simulink model "Australian14gen_forming_inertia"  (R2017b)
(part 2 of 4)

  T8/LConn2 -- B301/RConn2
  T8/RConn1 -- B303/LConn1
  T8/RConn2 -- B303/LConn2
  T8/RConn3 -- B303/LConn3
  B304/RConn1 -- L-23/LConn1 -- T10/LConn1
  B304/RConn2 -- L-23/LConn2 -- T10/LConn2
  T10/LConn3 -- L-23/LConn3 -- B304/RConn3
  L-33/LConn1 -- B314/RConn1
  L-33/LConn2 -- B314/RConn2
  L-33/LConn3 -- B314/RConn3
  L-33/RConn1 -- B313/LConn1
  L-33/RConn2 -- B313/LConn2
  L-33/RConn3 -- B313/LConn3
  T12/RConn3 -- Load17/LConn3 -- T22/RConn3 -- B314/LConn3
  T12/RConn2 -- T22/RConn2 -- Load17/LConn2 -- B314/LConn2
  T12/RConn1 -- T22/RConn1 -- Load17/LConn1 -- B314/LConn1
  T10/RConn1 -- B313/RConn1 -- Load16/LConn1 -- L-32/LConn1
  B313/RConn2 -- Load16/LConn2 -- L-32/LConn2 -- T10/RConn2
  T10/RConn3 -- B313/RConn3 -- Load16/LConn3 -- L-32/LConn3
  B312/LConn2 -- Load15/LConn2 -- L-32/RConn2
  L-32/RConn1 -- Load15/LConn1 -- B312/LConn1
  L-32/RConn3 -- Load15/LConn3 -- B312/LConn3
  G302_YPS/LConn3 -- B302/LConn3 -- Load Flow Bus11/LConn1
  T9/LConn3 -- B302/RConn3
  B312/RConn3 -- T18/RConn3 -- T9/RConn3
  T9/LConn2 -- B302/RConn2
  T9/LConn1 -- B302/RConn1
  B312/RConn2 -- T18/RConn2 -- T9/RConn2
  G302_YPS/LConn1 -- B302/LConn1
  G302_YPS/LConn2 -- B302/LConn2
  B312/RConn1 -- T18/RConn1 -- T9/RConn1
  B306/RConn1 -- L-26/LConn1 -- Load11/LConn1
  L-26/LConn2 -- Load11/LConn2 -- B306/RConn2
  B306/RConn3 -- L-26/LConn3 -- Load11/LConn3
  L-28/RConn1 -- B306/LConn1
  L-28/RConn2 -- B306/LConn2
  L-28/RConn3 -- B306/LConn3
  T11/RConn1 -- B311/LConn1
  T11/RConn2 -- B311/LConn2
  T11/RConn3 -- B311/LConn3
  B308/LConn1 -- Load13/LConn1 -- T13/LConn1
  B308/LConn2 -- Load13/LConn2 -- T13/LConn2
  B308/LConn3 -- Load13/LConn3 -- T13/LConn3
  T13/RConn1 -- B315/LConn1
  T13/RConn2 -- B315/LConn2
  T13/RConn3 -- B315/LConn3
  L-49-2/LConn1 -- B504/LConn1 -- L-48-1/LConn1 -- L-48-2/LConn1 -- L-49-1/LConn1
  L-49-2/LConn2 -- L-49-1/LConn2 -- L-48-1/LConn2 -- B504/LConn2 -- L-48-2/LConn2
  L-49-2/LConn3 -- L-49-1/LConn3 -- B504/LConn3 -- L-48-1/LConn3 -- L-48-2/LConn3
  B507/RConn2 -- Load27/LConn2 -- L-50-1/LConn2 -- L-48-2/RConn2 -- L-48-1/RConn2
  B507/RConn1 -- Load27/LConn1 -- L-48-2/RConn1 -- L-48-1/RConn1 -- L-50-1/LConn1
  B507/RConn3 -- Load27/LConn3 -- L-48-2/RConn3 -- L-48-1/RConn3 -- L-50-1/LConn3
  B509/RConn1 -- L-55-2/RConn1 -- L-55-1/RConn1
  B509/RConn2 -- L-55-2/RConn2 -- L-55-1/RConn2
  B509/RConn3 -- L-55-2/RConn3 -- L-55-1/RConn3
  L-55-2/LConn1 -- L-54/LConn1 -- L-55-1/LConn1 -- L-52/LConn1 -- B507/LConn1
  B507/LConn2 -- L-55-1/LConn2 -- L-52/LConn2 -- L-54/LConn2 -- L-55-2/LConn2
  L-54/LConn3 -- L-55-2/LConn3 -- B507/LConn3 -- L-55-1/LConn3 -- L-52/LConn3
  L-34-1/RConn1 -- L-34-2/RConn1 -- Three-Phase V-I Measurement4/RConn1
  L-34-1/RConn2 -- L-34-2/RConn2 -- Three-Phase V-I Measurement4/RConn2
  L-34-1/RConn3 -- L-34-2/RConn3 -- Three-Phase V-I Measurement4/RConn3
  B509/LConn1 -- Load29/LConn1 -- L-34-1/LConn1 -- L-34-2/LConn1
  Load29/LConn2 -- L-34-2/LConn2 -- L-34-1/LConn2 -- B509/LConn2
  B509/LConn3 -- L-34-1/LConn3 -- Load29/LConn3 -- L-34-2/LConn3
  G503_PPS/LConn3 -- Load Flow Bus12/LConn1 -- B503/LConn3
  G503_PPS/LConn1 -- B503/LConn1
  B503/RConn2 -- T21/LConn2
  B503/RConn3 -- T21/LConn3
  B503/RConn1 -- T21/LConn1
  G503_PPS/LConn2 -- B503/LConn2
  B506/RConn1 -- L-53/RConn1 -- L-52/RConn1
  B506/RConn2 -- L-53/RConn2 -- L-52/RConn2
  B506/RConn3 -- L-53/RConn3 -- L-52/RConn3
  B506/LConn2 -- T21/RConn2
  B506/LConn3 -- T21/RConn3
  B506/LConn1 -- T21/RConn1
  L-49-2/RConn1 -- L-49-1/RConn1 -- L-51/RConn1 -- L-54/RConn1 -- L-53/LConn1 -- B508/RConn1
  L-49-2/RConn2 -- L-49-1/RConn2 -- L-51/RConn2 -- L-54/RConn2 -- L-53/LConn2 -- B508/RConn2
  L-49-2/RConn3 -- L-49-1/RConn3 -- L-51/RConn3 -- L-54/RConn3 -- L-53/LConn3 -- B508/RConn3
  Load28/LConn1 -- T40/RConn1 -- T24/RConn1 -- B508/LConn1
  Load28/LConn2 -- T24/RConn2 -- T40/RConn2 -- B508/LConn2
  Load28/LConn3 -- T40/RConn3 -- T24/RConn3 -- B508/LConn3
  B505/RConn1 -- L-51/LConn1 -- L-50-1/RConn1
  B505/RConn2 -- L-51/LConn2 -- L-50-1/RConn2
  B505/RConn3 -- L-51/LConn3 -- L-50-1/RConn3
  B505/LConn3 -- T34/RConn3 -- T20/RConn3
  B502/RConn2 -- T20/LConn2
  B502/RConn1 -- T20/LConn1
  B505/LConn2 -- T34/RConn2 -- T20/RConn2
  B502/RConn3 -- T20/LConn3
  B505/LConn1 -- T34/RConn1 -- T20/RConn1
  B501/LConn2 -- T19/LConn2
  B501/LConn3 -- T19/LConn3
  B501/LConn1 -- T19/LConn1
  B504/RConn2 -- Load26/LConn2 -- T25/RConn2 -- T19/RConn2
  B504/RConn1 -- Load26/LConn1 -- T25/RConn1 -- T19/RConn1
  B504/RConn3 -- Load26/LConn3 -- T19/RConn3 -- T25/RConn3
  Load19/LConn1 -- B406/LConn1
  Load19/LConn2 -- B406/LConn2
  Load19/LConn3 -- B406/LConn3
  B204/LConn3 -- T5/LConn3
  G204_MPS/LConn1 -- Load Flow Bus8/LConn1 -- B204/RConn1
  G204_MPS/LConn3 -- B204/RConn3
  G204_MPS/LConn2 -- B204/RConn2
  B204/LConn1 -- T5/LConn1
  B204/LConn2 -- T5/LConn2
  B415/LConn1 -- Comp7-415/LConn1 -- L-47-2/LConn1 -- L-47-1/LConn1
  B415/LConn2 -- Comp7-415/LConn2 -- L-47-2/LConn2 -- L-47-1/LConn2
  B415/LConn3 -- Comp7-415/LConn3 -- L-47-2/LConn3 -- L-47-1/LConn3
  B416/RConn2 -- L-47-1/RConn2 -- L-47-2/RConn2
  B416/RConn3 -- L-47-1/RConn3 -- L-47-2/RConn3
  B416/RConn1 -- L-47-1/RConn1 -- L-47-2/RConn1
  B308/RConn1 -- T23/RConn1 -- L-29-1/LConn1 -- L-29-2/LConn1
  B308/RConn2 -- T23/RConn2 -- L-29-1/LConn2 -- L-29-2/LConn2
  B308/RConn3 -- T23/RConn3 -- L-29-1/LConn3 -- L-29-2/LConn3
  B307/LConn1 -- Load12/LConn1 -- L-29-1/RConn1 -- L-29-2/RConn1
  B307/LConn2 -- Load12/LConn2 -- L-29-1/RConn2 -- L-29-2/RConn2
  B307/LConn3 -- Load12/LConn3 -- L-29-1/RConn3 -- L-29-2/RConn3
  B205/RConn3 -- Three-Phase V-I Measurement1/RConn3
  B205/RConn2 -- Three-Phase V-I Measurement1/RConn2
  B205/RConn1 -- Three-Phase V-I Measurement1/RConn1
  L-30-2/LConn1 -- L-30-1/LConn1 -- B309/LConn1 -- Load14/LConn1
  2/RConn1 -- B310/LConn1 -- 1/RConn1
  1/RConn2 -- 2/RConn2 -- B310/LConn2
  2/RConn3 -- B310/LConn3 -- 1/RConn3
  2/LConn1 -- B311/RConn1 -- 1/LConn1
  2/LConn2 -- B311/RConn2 -- 1/LConn2
  1/LConn3 -- 2/LConn3 -- B311/RConn3
  L-2-1/RConn2 -- L-1-1/RConn2 -- L-1-2/RConn2 -- Three-Phase V-I Measurement2/LConn2 -- L-2-2/RConn2
  B102/RConn1 -- T27/RConn1 -- Three-Phase V-I Measurement2/RConn1
  B102/RConn2 -- T27/RConn2 -- Three-Phase V-I Measurement2/RConn2
  B102/RConn3 -- T27/RConn3 -- Three-Phase V-I Measurement2/RConn3
  L-30-1/RConn1 -- L-30-2/RConn1 -- B310/RConn1
  L-30-1/RConn2 -- L-30-2/RConn2 -- B310/RConn2
  L-30-1/RConn3 -- L-30-2/RConn3 -- B310/RConn3
  Three-Phase V-I Measurement3/RConn1 -- T26/RConn1 -- B309/RConn1
  Three-Phase V-I Measurement3/RConn2 -- T26/RConn2 -- B309/RConn2
  Three-Phase V-I Measurement3/RConn3 -- T26/RConn3 -- B309/RConn3
  B315/RConn3 -- Three-Phase V-I Measurement4/LConn3
  B315/RConn2 -- Three-Phase V-I Measurement4/LConn2
  B315/RConn1 -- Three-Phase V-I Measurement4/LConn1
  G404_GPS/LConn2 -- B404/RConn2
  G404_GPS/LConn1 -- B404/RConn1
  CPS403/LConn2 -- 20kV 2000MVA14/RConn2 -- 20kV 2000MVA1/RConn2 -- B403_vi/LConn2
  CPS403/LConn1 -- 20kV 2000MVA14/RConn1 -- 20kV 2000MVA1/RConn1 -- B403_vi/LConn1
  B402/LConn2 -- CPS402/LConn2
  CPS402/LConn3 -- B402/LConn3
  Load Flow Bus13/LConn1 -- 3-Phase Dynamic Load3/LConn3 -- B502/LConn3
  G501_NPS/LConn1 -- B501/RConn1
  B501/RConn2 -- G501_NPS/LConn2
  G501_NPS/LConn3 -- Load Flow Bus14/LConn1 -- B501/RConn3
  20kV 2000MVA8/RConn1 -- B312_vi/RConn1 -- 20kV 2000MVA19/RConn1
  20kV 2000MVA8/RConn2 -- B312_vi/RConn2 -- 20kV 2000MVA19/RConn2
  20kV 2000MVA8/RConn3 -- 20kV 2000MVA19/RConn3 -- B312_vi/RConn3
  B312_vi/LConn3 -- T18/LConn3
  T18/LConn2 -- B312_vi/LConn2
  T18/LConn1 -- B312_vi/LConn1
  B314_vi/LConn3 -- T22/LConn3
  20kV 2000MVA7/RConn2 -- 20kV 2000MVA20/RConn2 -- B314_vi/RConn2
  T22/LConn1 -- B314_vi/LConn1
  T22/LConn2 -- B314_vi/LConn2
  20kV 2000MVA7/RConn1 -- 20kV 2000MVA20/RConn1 -- B314_vi/RConn1
  20kV 2000MVA7/RConn3 -- 20kV 2000MVA20/RConn3 -- B314_vi/RConn3
  20kV 2000MVA10/RConn2 -- 20kV 2000MVA24/RConn2 -- B308_vi/LConn2
  T23/LConn2 -- B308_vi/RConn2
  T23/LConn3 -- B308_vi/RConn3
  20kV 2000MVA10/RConn1 -- 20kV 2000MVA24/RConn1 -- B308_vi/LConn1
  T23/LConn1 -- B308_vi/RConn1
  20kV 2000MVA10/RConn3 -- 20kV 2000MVA24/RConn3 -- B308_vi/LConn3
  B508_vi/LConn3 -- 20kV 2000MVA26/RConn1 -- 20kV 2000MVA13/RConn1
  B508_vi/LConn2 -- 20kV 2000MVA26/RConn2 -- 20kV 2000MVA13/RConn2
  B508_vi/LConn1 -- 20kV 2000MVA26/RConn3 -- 20kV 2000MVA13/RConn3
  T25/LConn3 -- B504_vi/RConn3
  T25/LConn1 -- B504_vi/RConn1
  T25/LConn2 -- B504_vi/RConn2
  20kV 2000MVA11/RConn1 -- 20kV 2000MVA27/RConn1 -- B504_vi/LConn1
  20kV 2000MVA11/RConn2 -- 20kV 2000MVA27/RConn2 -- B504_vi/LConn2
  20kV 2000MVA11/RConn3 -- 20kV 2000MVA27/RConn3 -- B504_vi/LConn3
  B508_vi/RConn3 -- T24/LConn1
  T24/LConn2 -- B508_vi/RConn2
  B508_vi/RConn1 -- T24/LConn3
  20kV 2000MVA9/RConn1 -- 20kV 2000MVA25/RConn1 -- B309_vi/RConn3
  20kV 2000MVA9/RConn2 -- 20kV 2000MVA25/RConn2 -- B309_vi/RConn2
  20kV 2000MVA9/RConn3 -- 20kV 2000MVA25/RConn3 -- B309_vi/RConn1
  T26/LConn1 -- B309_vi/LConn3
  T26/LConn2 -- B309_vi/LConn2
  T26/LConn3 -- B309_vi/LConn1
  B102_vi/LConn1 -- T27/LConn1
  B102_vi/LConn2 -- T27/LConn2
  B102_vi/LConn3 -- T27/LConn3
  15kV 1500MVA11/RConn1 -- 20kV 2000MVA18/RConn1 -- B102_vi/RConn1
  15kV 1500MVA11/RConn2 -- 20kV 2000MVA18/RConn2 -- B102_vi/RConn2
  15kV 1500MVA11/RConn3 -- 20kV 2000MVA18/RConn3 -- B102_vi/RConn3
  B212_vi/LConn1 -- T28/LConn1
  T28/LConn2 -- B212_vi/LConn2
  B212_vi/LConn3 -- T28/LConn3
  20kV 2000MVA4/RConn1 -- 20kV 2000MVA17/RConn1 -- B212_vi/RConn1
  20kV 2000MVA4/RConn2 -- 20kV 2000MVA17/RConn2 -- B212_vi/RConn2
  20kV 2000MVA4/RConn3 -- 20kV 2000MVA17/RConn3 -- B212_vi/RConn3
  20kV 2000MVA5/RConn1 -- 20kV 2000MVA22/RConn1 -- B216_vi/LConn1
  20kV 2000MVA5/RConn2 -- 20kV 2000MVA22/RConn2 -- B216_vi/LConn2
  20kV 2000MVA5/RConn3 -- B216_vi/LConn3 -- 20kV 2000MVA22/RConn3
  T29/LConn1 -- B216_vi/RConn1
  T29/LConn2 -- B216_vi/RConn2
  T29/LConn3 -- B216_vi/RConn3
  20kV 2000MVA6/RConn1 -- 20kV 2000MVA23/RConn1 -- B215_vi/RConn1
  20kV 2000MVA6/RConn2 -- 20kV 2000MVA23/RConn2 -- B215_vi/RConn2
  20kV 2000MVA6/RConn3 -- 20kV 2000MVA23/RConn3 -- B215_vi/RConn3
  T30/LConn1 -- B215_vi/LConn1
  T30/LConn2 -- B215_vi/LConn2
  T30/LConn3 -- B215_vi/LConn3
  T31/LConn1 -- B208_vi/LConn1
  T31/LConn2 -- B208_vi/LConn2
  T31/LConn3 -- B208_vi/LConn3
  T32/LConn1 -- B410_vi/RConn1
  T32/LConn2 -- B410_vi/RConn2
  T32/LConn3 -- B410_vi/RConn3
  T33/LConn1 -- B405_vi/LConn1
  T33/LConn2 -- B405_vi/LConn2
  T33/LConn3 -- B405_vi/LConn3
  T34/LConn1 -- B502_vi/RConn1
  T34/LConn2 -- B502_vi/RConn2
  T34/LConn3 -- B502_vi/RConn3
  20kV 2000MVA12/RConn1 -- 20kV 2000MVA28/RConn1 -- B502_vi/LConn1
  20kV 2000MVA12/RConn2 -- 20kV 2000MVA28/RConn2 -- B502_vi/LConn2
  20kV 2000MVA12/RConn3 -- 20kV 2000MVA28/RConn3 -- B502_vi/LConn3
  Dist410/RConn1 -- T35/LConn1
  Dist410/RConn2 -- T35/LConn2
  Dist410/RConn3 -- T35/LConn3
  T36/LConn1 -- Dist411/RConn1
  T36/LConn2 -- Dist411/RConn2
  T36/LConn3 -- Dist411/RConn3
  T37/LConn1 -- Dist206/RConn1
  T37/LConn3 -- Dist206/RConn3
  T37/LConn2 -- Dist206/RConn2
  T38/LConn1 -- Dist212/RConn1
  T38/LConn2 -- Dist212/RConn2
  T38/LConn3 -- Dist212/RConn3
  T39/LConn1 -- Dist307/RConn1
  T39/LConn2 -- Dist307/RConn2
  T39/LConn3 -- Dist307/RConn3
  T40/LConn1 -- Dist508/RConn1
  T40/LConn2 -- Dist508/RConn2
  T40/LConn3 -- Dist508/RConn3
  3-Phase Dynamic Load3/LConn1 -- B502/LConn1
  B502/LConn2 -- 3-Phase Dynamic Load3/LConn2
  20kV 2000MVA/LConn1 -- fake_VSC_410/RConn1 -- INV410/LConn1
  20kV 2000MVA/LConn2 -- fake_VSC_410/RConn2 -- INV410/LConn2
  20kV 2000MVA/LConn3 -- Load Flow Bus16/LConn1 -- fake_VSC_410/RConn3 -- INV410/LConn3
  20kV 2000MVA/RConn1 -- 20kV 2000MVA21/RConn1 -- B410_vi/LConn1
  20kV 2000MVA/RConn2 -- 20kV 2000MVA21/RConn2 -- B410_vi/LConn2
  20kV 2000MVA/RConn3 -- 20kV 2000MVA21/RConn3 -- B410_vi/LConn3
  20kV 2000MVA1/LConn1 -- fake_VSC_403/RConn1 -- INV403/LConn1
  20kV 2000MVA1/LConn3 -- Load Flow Bus1/LConn1 -- fake_VSC_403/RConn3 -- INV403/LConn3
  20kV 2000MVA1/LConn2 -- fake_VSC_403/RConn2 -- INV403/LConn2
  20kV 2000MVA2/LConn1 -- fake_VSC_405/RConn1 -- INV405/LConn1
  20kV 2000MVA2/LConn3 -- Load Flow Bus29/LConn1 -- fake_VSC_405/RConn3 -- INV405/LConn3
  20kV 2000MVA2/LConn2 -- fake_VSC_405/RConn2 -- INV405/LConn2
  20kV 2000MVA2/RConn1 -- 20kV 2000MVA15/RConn1 -- B405_vi/RConn1
  20kV 2000MVA2/RConn2 -- 20kV 2000MVA15/RConn2 -- B405_vi/RConn2
  20kV 2000MVA2/RConn3 -- 20kV 2000MVA15/RConn3 -- B405_vi/RConn3
  20kV 2000MVA3/LConn2 -- fake_VSC_208/RConn2 -- INV208/LConn2
  20kV 2000MVA3/LConn1 -- fake_VSC_208/RConn1 -- INV208/LConn1
  20kV 2000MVA3/LConn3 -- fake_VSC_208/RConn3 -- Load Flow Bus28/LConn1 -- INV208/LConn3
  20kV 2000MVA3/RConn1 -- 20kV 2000MVA16/RConn1 -- B208_vi/RConn1
  20kV 2000MVA3/RConn2 -- 20kV 2000MVA16/RConn2 -- B208_vi/RConn2
  20kV 2000MVA3/RConn3 -- 20kV 2000MVA16/RConn3 -- B208_vi/RConn3
  20kV 2000MVA4/LConn2 -- INV212/LConn2 -- fake_VSC_212/RConn2
  20kV 2000MVA4/LConn1 -- INV212/LConn1 -- fake_VSC_212/RConn1
  20kV 2000MVA4/LConn3 -- Load Flow Bus27/LConn1 -- INV212/LConn3 -- fake_VSC_212/RConn3
  20kV 2000MVA5/LConn2 -- fake_VSC_216/RConn2 -- INV216/LConn2
  20kV 2000MVA5/LConn1 -- fake_VSC_216/RConn1 -- Load Flow Bus25/LConn1 -- INV216/LConn1
  20kV 2000MVA5/LConn3 -- fake_VSC_216/RConn3 -- INV216/LConn3
  INV215/LConn1 -- Load Flow Bus26/LConn1 -- 20kV 2000MVA6/LConn1 -- fake_VSC_215/RConn1
  INV215/LConn2 -- 20kV 2000MVA6/LConn2 -- fake_VSC_215/RConn2
  INV215/LConn3 -- 20kV 2000MVA6/LConn3 -- fake_VSC_215/RConn3
  20kV 2000MVA7/LConn2 -- fake_VSC_314/RConn2 -- INV314/LConn2
  20kV 2000MVA7/LConn1 -- fake_VSC_314/RConn1 -- INV314/LConn1
  20kV 2000MVA7/LConn3 -- Load Flow Bus21/LConn1 -- fake_VSC_314/RConn3 -- INV314/LConn3
  20kV 2000MVA8/LConn2 -- fake_VSC_312/RConn2 -- INV312/LConn2
  20kV 2000MVA8/LConn1 -- Load Flow Bus22/LConn1 -- INV312/LConn1 -- fake_VSC_312/RConn1
  20kV 2000MVA8/LConn3 -- fake_VSC_312/RConn3 -- INV312/LConn3
  20kV 2000MVA9/LConn2 -- fake_VSC_309/RConn2 -- INV309/LConn2
  20kV 2000MVA9/LConn1 -- Load Flow Bus23/LConn1 -- fake_VSC_309/RConn1 -- INV309/LConn1
  20kV 2000MVA9/LConn3 -- fake_VSC_309/RConn3 -- INV309/LConn3
  20kV 2000MVA10/LConn2 -- fake_VSC_308/RConn2 -- INV308/LConn2
  20kV 2000MVA10/LConn1 -- INV308/LConn1 -- fake_VSC_308/RConn1
  20kV 2000MVA10/LConn3 -- Load Flow Bus20/LConn1 -- fake_VSC_308/RConn3 -- INV308/LConn3
  15kV 1500MVA11/LConn2 -- fake_VSC_2/RConn2 -- INV102/LConn2
  15kV 1500MVA11/LConn1 -- Load Flow Bus24/LConn1 -- fake_VSC_2/RConn1 -- INV102/LConn1
  15kV 1500MVA11/LConn3 -- fake_VSC_2/RConn3 -- INV102/LConn3
  20kV 2000MVA11/LConn3 -- fake_VSC_504/RConn3 -- INV504/LConn3
  20kV 2000MVA11/LConn2 -- fake_VSC_504/RConn2 -- INV504/LConn2
  20kV 2000MVA11/LConn1 -- fake_VSC_504/RConn1 -- INV504/LConn1 -- Load Flow Bus17/LConn1
  20kV 2000MVA12/LConn3 -- Load Flow Bus18/LConn1 -- fake_VSC_502/RConn3 -- INV502/LConn3
  20kV 2000MVA12/LConn2 -- fake_VSC_502/RConn2 -- INV502/LConn2
  20kV 2000MVA12/LConn1 -- fake_VSC_502/RConn1 -- INV502/LConn1
  20kV 2000MVA13/LConn3 -- Load Flow Bus19/LConn1 -- fake_VSC_508/RConn3 -- INV508/LConn3
  20kV 2000MVA13/LConn2 -- fake_VSC_508/RConn2 -- INV508/LConn2
  20kV 2000MVA13/LConn1 -- fake_VSC_508/RConn1 -- INV508/LConn1
  20kV 2000MVA14/LConn1 -- Ground/LConn1 -- 20kV 2000MVA14/LConn2 -- 20kV 2000MVA14/LConn3
  20kV 2000MVA15/LConn1 -- Ground1/LConn1 -- 20kV 2000MVA15/LConn2 -- 20kV 2000MVA15/LConn3
  20kV 2000MVA16/LConn1 -- Ground2/LConn1 -- 20kV 2000MVA16/LConn2 -- 20kV 2000MVA16/LConn3
  20kV 2000MVA17/LConn1 -- Ground3/LConn1 -- 20kV 2000MVA17/LConn2 -- 20kV 2000MVA17/LConn3
  20kV 2000MVA18/LConn1 -- Ground4/LConn1 -- 20kV 2000MVA18/LConn2 -- 20kV 2000MVA18/LConn3
  20kV 2000MVA19/LConn1 -- Ground5/LConn1 -- 20kV 2000MVA19/LConn3 -- 20kV 2000MVA19/LConn2
  20kV 2000MVA20/LConn1 -- Ground6/LConn1 -- 20kV 2000MVA20/LConn2 -- 20kV 2000MVA20/LConn3
  20kV 2000MVA21/LConn1 -- Ground7/LConn1 -- 20kV 2000MVA21/LConn2 -- 20kV 2000MVA21/LConn3
  20kV 2000MVA22/LConn1 -- 20kV 2000MVA22/LConn3 -- Ground8/LConn1 -- 20kV 2000MVA22/LConn2
  20kV 2000MVA23/LConn1 -- Ground9/LConn1 -- 20kV 2000MVA23/LConn2 -- 20kV 2000MVA23/LConn3
  20kV 2000MVA24/LConn1 -- 20kV 2000MVA24/LConn2 -- Ground10/LConn1 -- 20kV 2000MVA24/LConn3
  20kV 2000MVA25/LConn1 -- Ground11/LConn1 -- 20kV 2000MVA25/LConn3 -- 20kV 2000MVA25/LConn2
  20kV 2000MVA26/LConn1 -- Ground12/LConn1 -- 20kV 2000MVA26/LConn3 -- 20kV 2000MVA26/LConn2
  20kV 2000MVA27/LConn1 -- Ground13/LConn1 -- 20kV 2000MVA27/LConn2 -- 20kV 2000MVA27/LConn3
  20kV 2000MVA28/LConn1 -- Ground14/LConn1 -- 20kV 2000MVA28/LConn2 -- 20kV 2000MVA28/LConn3
  Three-Phase V-I Measurement5/LConn1 -- 3-Phase Dynamic Load4/LConn1
  Three-Phase V-I Measurement5/LConn2 -- 3-Phase Dynamic Load4/LConn2
  Three-Phase V-I Measurement5/LConn3 -- 3-Phase Dynamic Load4/LConn3
  Three-Phase V-I Measurement5/RConn1 -- B101/RConn1
  Three-Phase V-I Measurement5/RConn2 -- B101/RConn2
